simulink model "SystemModel"  (R2017b)
settings: Solver=VariableStepAuto  StartTime=0.0  StopTime=10.0  RelTol=1e-3
settings Model: Creator=rarora  LastModifiedBy=rarora

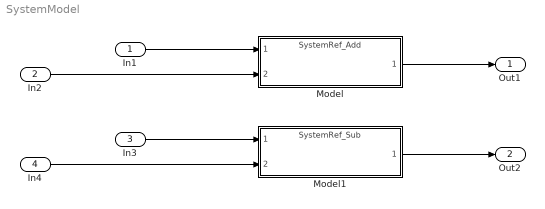
== system SystemModel ==
  In1 : Inport
  In2 : Inport  Port=2
  In3 : Inport  Port=3
  In4 : Inport  Port=4
  Model : ModelReference  ModelNameDialog=SystemRef_Add.slx  SimulationMode=Normal  ModelReferenceVersion=1.1
  Model1 : ModelReference  ModelNameDialog=SystemRef_Sub.slx  SimulationMode=Normal  ModelReferenceVersion=1.1
  Out1 : Outport
  Out2 : Outport  Port=2
  wires:
  In2/1 -> Model/2
  In1/1 -> Model/1
  In3/1 -> Model1/1
  In4/1 -> Model1/2
  Model/1 -> Out1/1
  Model1/1 -> Out2/1
